simulink model "THEIA_EPS"  (R2024b)
settings: Solver=FixedStepDiscrete  StartTime=0.0  StopTime=60  RelTol=1e-3
undefined symbols (not defined in the file or in its folder): Ion, Lithium
libraries: spsSeriesRLCBranchLib x7, spsIGBTDiodeLib x3, spsIdealSwitchLib x2, slpidlib x2, spsPWMGeneratorDCDCLib x2, spsBatteryLib x1, spsCurrentMeasurementLib x1, spsDiodeLib x1, spsPVArrayLib x1, spsVoltageMeasurementLib x1, sps_lib x1
settings Model: SimulationMode=accelerator  Creator=Josh  LastModifiedBy=Josh

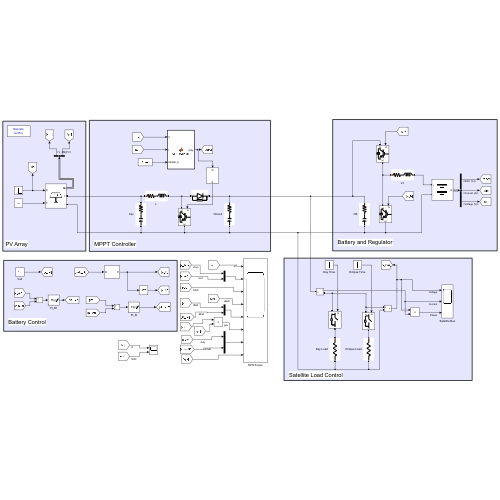
[thumbnail: Simulink's stored preview of the top-level diagram]
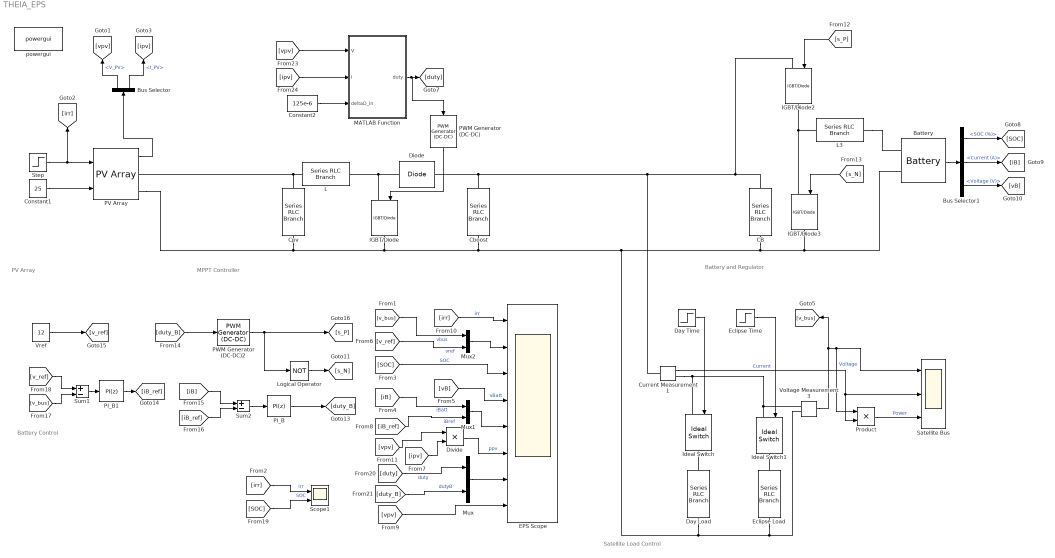
== system THEIA_EPS ==
  note: Battery Control
  note: Satellite Load Control
  note: Battery and Regulator
  note: MPPT Controller
  note: PV Array
  Battery : spsBatteryLib/Battery  BatType=Lithium-Ion  NomV=8  NomQ=12.5  SOC=80  Batt_Tr=1  PresetModel=on  MaxQ=12.5  MinV=6  FullV=9.3119  Dis_rate=5.4348  R=0.0064  Normal_OP=11.3043  expZone="[8.6431     0.61413]"
  Bus Selector : BusSelector  OutputSignals=V_PV,I_PV
  Bus Selector1 : BusSelector  OutputSignals=SOC (%),Current (A),Voltage (V)
  CB : spsSeriesRLCBranchLib/Series RLC Branch  LConnTagsString=__new0  RConnTagsString=__new0  BranchType=RC  Resistance=1e-4  Inductance=1e-3  SetiL0=off  InitialCurrent=0  Capacitance=1000e-6  Setx0=off  InitialVoltage=0  Measurements=None
  Cboost : spsSeriesRLCBranchLib/Series RLC Branch  LConnTagsString=__new0  RConnTagsString=__new0  BranchType=RC  Resistance=1e-4  Inductance=1e-3  SetiL0=off  InitialCurrent=0  Capacitance=3300e-6  Setx0=off  InitialVoltage=0  Measurements=None
  Constant1 : Constant  Value=25
  Constant2 : Constant  Value=125e-6
  Cpv : spsSeriesRLCBranchLib/Series RLC Branch  LConnTagsString=__new0  RConnTagsString=__new0  BranchType=RC  Resistance=1e-4  Inductance=1e-3  SetiL0=off  InitialCurrent=0  Capacitance=100e-6  Setx0=off  InitialVoltage=0  Measurements=None
  Current Measurement1 : spsCurrentMeasurementLib/Current Measurement  PhasorSimulation=off  OutputType=Complex  PSBequivalent=0
  Day Load : spsSeriesRLCBranchLib/Series RLC Branch  LConnTagsString=__new0  RConnTagsString=__new0  BranchType=R  Resistance=1.7  Inductance=5e-3  SetiL0=off  InitialCurrent=0  Capacitance=100e-6  Setx0=off  InitialVoltage=0  Measurements=None
  Day Time : Step  Time=30  Before=1  After=0  SampleTime=0
  Diode : spsDiodeLib/Diode  Ron=0.001  Lon=0  Vf=0.8  IC=0  UseSnubber=0  Rs=5000  Cs=250e-9  Measurements=off
  Divide : Product  Inputs=**
  EPS Scope : Scope  NumInputPorts=8
  Eclipse Load : spsSeriesRLCBranchLib/Series RLC Branch  LConnTagsString=__new0  RConnTagsString=__new0  BranchType=R  Resistance=31  Inductance=5e-3  SetiL0=off  InitialCurrent=0  Capacitance=100e-6  Setx0=off  InitialVoltage=0  Measurements=None
  Eclipse Time : Step  Time=30  SampleTime=0
  IGBT/Diode : spsIGBTDiodeLib/IGBT//Diode  Ron=1e-3  Rs=1e5  Cs=inf  Measurements=off
  IGBT/Diode2 : spsIGBTDiodeLib/IGBT//Diode  Ron=1e-3  Rs=1e5  Cs=inf  Measurements=off
  IGBT/Diode3 : spsIGBTDiodeLib/IGBT//Diode  Ron=1e-3  Rs=1e5  Cs=inf  Measurements=off
  Ideal Switch : spsIdealSwitchLib/Ideal Switch  Ron=0.001  Lon=0  IC=0  Rs=1e5  Cs=inf  Measurements=off
  Ideal Switch1 : spsIdealSwitchLib/Ideal Switch  Ron=0.001  Lon=0  IC=0  Rs=1e5  Cs=inf  Measurements=off
  L : spsSeriesRLCBranchLib/Series RLC Branch  LConnTagsString=__new0  RConnTagsString=__new0  BranchType=RL  Resistance=0.1  Inductance=5e-3  SetiL0=off  InitialCurrent=0  Capacitance=100e-6  Setx0=off  InitialVoltage=0  Measurements=None
  L3 : spsSeriesRLCBranchLib/Series RLC Branch  LConnTagsString=__new0  RConnTagsString=__new0  BranchType=RL  Resistance=0.1  Inductance=5e-3  SetiL0=off  InitialCurrent=0  Capacitance=100e-6  Setx0=off  InitialVoltage=0  Measurements=None
  Logical Operator : Logic  Operator=NOT  AllPortsSameDT=off  OutDataTypeStr=boolean
  MATLAB Function : MATLAB Function  TreatAsAtomicUnit=on
  Mux : Mux  Inputs=2
  Mux1 : Mux  Inputs=2
  Mux2 : Mux  Inputs=2
  PI_B : slpidlib/PID Controller  Controller=PI  Form=Parallel  TimeDomain=Discrete-time  UseExternalTs=off  SampleTime=50e-6  IntegratorMethod=Forward Euler  FilterMethod=Forward Euler  ControllerParametersSource=internal  P=0.02  I=10  UseKiTs=off  D=1e-4  UseExternalDerivativeSource=off  N=100  UseFilter=off  TunerSelectOption=Transfer Function Based (PID Tuner App)  InitialConditionSource=internal  InitialConditionForIntegrator=0  InitialConditionForFilter=0  DifferentiatorICPrevScaledInput=0  ExternalReset=none  TrackingMode=off  Kt=1  LimitOutput=on  SatLimitsSource=internal  UpperSaturationLimit=0.95  LowerSaturationLimit=0  LinearizeAsGain=off  AntiWindupMode=none  Kb=1  LimitIntegrator=off  UpperIntegratorSaturationLimit=inf  LowerIntegratorSaturationLimit=-inf  POutMin=[]  POutMax=[]  IOutMin=[]  IOutMax=[]  DOutMin=[]  DOutMax=[]  NOutMin=[]  NOutMax=[]  SumOutMin=[]  SumOutMax=[]  SaturationOutMin=[]  SaturationOutMax=[]  PParamMin=[]  PParamMax=[]  IParamMin=[]  IParamMax=[]  DParamMin=[]  DParamMax=[]  NParamMin=[]  NParamMax=[]  KbParamMin=[]  KbParamMax=[]  KtParamMin=[]  KtParamMax=[]  KbOutMin=[]  KbOutMax=[]  KtOutMin=[]  KtOutMax=[]  IntegratorOutMin=[]  IntegratorOutMax=[]  FilterOutMin=[]  FilterOutMax=[]  SumI1OutMin=[]  SumI1OutMax=[]  SumI2OutMin=[]  SumI2OutMax=[]  SumI3OutMin=[]  SumI3OutMax=[]  SumI4OutMin=[]  SumI4OutMax=[]  SumDOutMin=[]  SumDOutMax=[]  DifferentiatorOutMin=[]  DifferentiatorOutMax=[]  FilterDiffOutCoefMin=[]  FilterDiffOutCoefMax=[]  ReciprocalOutMin=[]  ReciprocalOutMax=[]  SumDenOutMin=[]  SumDenOutMax=[]  SumNumOutMin=[]  SumNumOutMax=[]  DivideOutMin=[]  DivideOutMax=[]  UdiffTsProdOutMin=[]  UdiffTsProdOutMax=[]  NTsProdOutMin=[]  NTsProdOutMax=[]  UintegralTsProdOutMin=[]  UintegralTsProdOutMax=[]  UngainTsProdOutMin=[]  UngainTsProdOutMax=[]  ClampingZeroOutDataTypeStr=Inherit: Inherit via back propagation  ClampingZeroOutMin=[]  ClampingZeroOutMax=[]  FilterDenConstantOutDataTypeStr=Inherit: Inherit via back propagation  FilterDenConstantOutMin=[]  FilterDenConstantOutMax=[]  PCopyOutDataTypeStr=Inherit: Inherit via back propagation  PCopyOutMin=[]  PCopyOutMax=[]  NCopyOutDataTypeStr=Inherit: Inherit via back propagation  NCopyOutMin=[]  NCopyOutMax=[]  IntegratorContinuousStateAttributes=''  IntegratorStateMustResolveToSignalObject=off  IntegratorRTWStateStorageClass=Auto  FilterContinuousStateAttributes=''  FilterStateMustResolveToSignalObject=off  FilterRTWStateStorageClass=Auto  ParallelPVariant=InternalParameters  IdealPVariant=Disabled  IVariant=InternalParameters  DVariant=Disabled  IntegratorVariant=Discrete  SatVariant=Enabled  AWVariant=Passthrough  PCopyVariant=Disabled  TRVariant=Disabled  FdbkBlocksVariant=Forward  IdealPFdbkVariant=Disabled  SatFdbkVariant=Disabled  DerivativeFilterVariant=Disabled  NVariant=Disabled  NCopyVariant=Disabled_SignalSpec  FilterICVariant=Disabled  IntegratorICVariant=InternalICs  ExternalResetVariant=Disabled  TRSumVariant=Passthrough  SumFdbkVariant=Disabled  SumVariant=Sum_PI  TsampFilterVariant=InternalTs  TsampNgainVariant=Passthrough  TsampIntegralVariant=Disabled_SignalSpec  ExternalSaturationOutDataTypeStr=Inherit: Same as second input  DerivativeSourceVariant=Disabled  PreIntVariant=InternalPreInt
      settings: LibrarySourceBlock=simulink/Discrete/Discrete PID Controller
  PI_B1 : slpidlib/PID Controller  Controller=PI  Form=Parallel  TimeDomain=Discrete-time  UseExternalTs=off  SampleTime=500e-6  IntegratorMethod=Forward Euler  FilterMethod=Forward Euler  ControllerParametersSource=internal  P=0.8  I=5  UseKiTs=off  D=10  UseExternalDerivativeSource=off  N=100  UseFilter=on  TunerSelectOption=Frequency Response Based  InitialConditionSource=internal  InitialConditionForIntegrator=0  InitialConditionForFilter=0  DifferentiatorICPrevScaledInput=0  ExternalReset=none  TrackingMode=off  Kt=1  LimitOutput=on  SatLimitsSource=internal  UpperSaturationLimit=5.5  LowerSaturationLimit=-5.5  LinearizeAsGain=off  AntiWindupMode=none  Kb=1  LimitIntegrator=off  UpperIntegratorSaturationLimit=inf  LowerIntegratorSaturationLimit=-inf  POutMin=[]  POutMax=[]  IOutMin=[]  IOutMax=[]  DOutMin=[]  DOutMax=[]  NOutMin=[]  NOutMax=[]  SumOutMin=[]  SumOutMax=[]  SaturationOutMin=[]  SaturationOutMax=[]  PParamMin=[]  PParamMax=[]  IParamMin=[]  IParamMax=[]  DParamMin=[]  DParamMax=[]  NParamMin=[]  NParamMax=[]  KbParamMin=[]  KbParamMax=[]  KtParamMin=[]  KtParamMax=[]  KbOutMin=[]  KbOutMax=[]  KtOutMin=[]  KtOutMax=[]  IntegratorOutMin=[]  IntegratorOutMax=[]  FilterOutMin=[]  FilterOutMax=[]  SumI1OutMin=[]  SumI1OutMax=[]  SumI2OutMin=[]  SumI2OutMax=[]  SumI3OutMin=[]  SumI3OutMax=[]  SumI4OutMin=[]  SumI4OutMax=[]  SumDOutMin=[]  SumDOutMax=[]  DifferentiatorOutMin=[]  DifferentiatorOutMax=[]  FilterDiffOutCoefMin=[]  FilterDiffOutCoefMax=[]  ReciprocalOutMin=[]  ReciprocalOutMax=[]  SumDenOutMin=[]  SumDenOutMax=[]  SumNumOutMin=[]  SumNumOutMax=[]  DivideOutMin=[]  DivideOutMax=[]  UdiffTsProdOutMin=[]  UdiffTsProdOutMax=[]  NTsProdOutMin=[]  NTsProdOutMax=[]  UintegralTsProdOutMin=[]  UintegralTsProdOutMax=[]  UngainTsProdOutMin=[]  UngainTsProdOutMax=[]  ClampingZeroOutDataTypeStr=Inherit: Inherit via back propagation  ClampingZeroOutMin=[]  ClampingZeroOutMax=[]  FilterDenConstantOutDataTypeStr=Inherit: Inherit via back propagation  FilterDenConstantOutMin=[]  FilterDenConstantOutMax=[]  PCopyOutDataTypeStr=Inherit: Inherit via back propagation  PCopyOutMin=[]  PCopyOutMax=[]  NCopyOutDataTypeStr=Inherit: Inherit via back propagation  NCopyOutMin=[]  NCopyOutMax=[]  IntegratorContinuousStateAttributes=''  IntegratorStateMustResolveToSignalObject=off  IntegratorRTWStateStorageClass=Auto  FilterContinuousStateAttributes=''  FilterStateMustResolveToSignalObject=off  FilterRTWStateStorageClass=Auto  ParallelPVariant=InternalParameters  IdealPVariant=Disabled  IVariant=InternalParameters  DVariant=Disabled  IntegratorVariant=Discrete  SatVariant=Enabled  AWVariant=Passthrough  PCopyVariant=Disabled  TRVariant=Disabled  FdbkBlocksVariant=Forward  IdealPFdbkVariant=Disabled  SatFdbkVariant=Disabled  DerivativeFilterVariant=Disabled  NVariant=Disabled  NCopyVariant=Disabled_SignalSpec  FilterICVariant=Disabled  IntegratorICVariant=InternalICs  ExternalResetVariant=Disabled  TRSumVariant=Passthrough  SumFdbkVariant=Disabled  SumVariant=Sum_PI  TsampFilterVariant=InternalTs  TsampNgainVariant=Passthrough  TsampIntegralVariant=Disabled_SignalSpec  ExternalSaturationOutDataTypeStr=Inherit: Same as second input  DerivativeSourceVariant=Disabled  PreIntVariant=InternalPreInt
      settings: LibrarySourceBlock=simulink/Discrete/Discrete PID Controller
  PV Array : spsPVArrayLib/PV Array  Npar=18  Nser=1  PlotType=array @ 25 deg.C & specified irradiances  S_vec=[1367 1000 500 0]  Temp_C_vec="[ 45 25  ]"  ModuleName=User-defined  PlotWhenSelected=off  Pm=5.0021  Ncell=7  Voc=17.136  Isc=0.342  Vm=15.1578  Im=0.33  beta_Voc_pc=-0.2369  alpha_Isc_pc=0.0022  beta_Voc=-0.040595  alpha_Isc=7.524e-06  IL=0.34471  I0=5.8844e-14  nI=3.2418  Rsh=7127.5853  Rs=0.16891  RobustModel=off  RobustCellTemperature=313.3991  BAL=on  Tc=1e-6  Tfilter=5e-5
  PWM Generator (DC-DC) : spsPWMGeneratorDCDCLib/PWM Generator (DC-DC)  Fsw=5000  Ts=10e-6
  PWM Generator (DC-DC)2 : spsPWMGeneratorDCDCLib/PWM Generator (DC-DC)  Fsw=5000  Ts=10e-6
  Product : Product
  Satellite Bus : Scope  NumInputPorts=3
  Scope1 : Scope  NumInputPorts=2
  Step : Step  Time=30  Before=1367  After=0  SampleTime=0
  Sum1 : Sum  Inputs=+-
  Sum2 : Sum  Inputs=+-
  Voltage Measurement3 : spsVoltageMeasurementLib/Voltage Measurement  PhasorSimulation=off  OutputType=Complex  PSBequivalent=0
  Vref : Constant  Value=12
  powergui : sps_lib/powergui  Priority=1  SimulationMode=Discrete  SampleTime=10e-6  frequency=60  Iterations=50  frequencyindice=0  Pbase=100e6  ErrMax=1e-4  UnitsV=kV  UnitsW=MW  buscounter=0  FunctionMessages=off  echomessages=off  EnableUseOfTLC=off  CurrentSourceSwitches=off  DisableSnubberDevices=off  DisableRonSwitches=off  DisableVfSwitches=off  DisplayEquations=off  AutomaticDiscreteSolvers=off  SolverType=Tustin/Backward Euler (TBE)  Interpol=off  ExternalGateDelay=off  methode=off  Ts=100  x0status=blocks  SPID=on  SwTol=0  HookPort=off  NonlinearTolerance=1e-4  nMaxIteration=100  ContinueOnMaxIteration=off  RestoreLinks=warning  ResistiveCurrentMeasurement=off  Frange=[0:2:500]  Ylog=off  Xlog=on  ShowGrid=off  save=off  variable=ZData  structure=0  ZoomFFT=off  StartTime=0.0  cycles=1  DisplayStyle=1  fundamental=60  FreqAxis=off  MaxFrequency=1000  frequencyindicesteady=1  RmsSteady=1  display=off
  wires:
  Constant1/1 -> PV Array/2
  Step/1 -> [irr], PV Array/1
  Constant2/1 -> MATLAB Function/3(deltaD_in)
  MATLAB Function/1(duty) -> PWM Generator (DC-DC)/1, [duty]
  PWM Generator (DC-DC)/1 -> IGBT/Diode/1
  PWM Generator (DC-DC)2/1 -> Logical Operator/1, [s_P]
  Sum2/1 -> PI_B/1
  Vref/1 -> [v_ref]
  PI_B1/1 -> [iB_ref]
  [duty_B] -> PWM Generator (DC-DC)2/1
  PI_B/1 -> [duty_B]
  Sum1/1 -> PI_B1/1
  [s_P] -> IGBT/Diode2/1
  Battery/1 -> Bus Selector1/1
  [s_N] -> IGBT/Diode3/1
  Bus Selector1/1 -> [SOC]  "<SOC (%)>"
  Bus Selector1/2 -> [iB]  "<Current (A)>"
  Bus Selector1/3 -> [vB]  "<Voltage (V)>"
  [vB] -> EPS Scope/4  "vBatt"
  [irr] -> EPS Scope/1  "irr"
  Mux1/1 -> EPS Scope/5
  [iB] -> Mux1/1  "iBatt"
  [iB_ref] -> Mux1/2  "iBref"
  Mux2/1 -> EPS Scope/2
  [v_bus] -> Mux2/1  "vbus"
  [v_ref] -> Mux2/2  "vref"
  [SOC] -> EPS Scope/3  "SOC"
  [ipv] -> Divide/2
  [vpv] -> Divide/1
  Divide/1 -> EPS Scope/6  "ppv"
  PV Array/1 -> Bus Selector/1
  Bus Selector/2 -> [ipv]  "<I_PV>"
  Bus Selector/1 -> [vpv]  "<V_PV>"
  Mux/1 -> EPS Scope/7
  [duty] -> Mux/1  "duty"
  [duty_B] -> Mux/2  "dutyB"
  [v_ref] -> Sum1/1
  [v_bus] -> Sum1/2
  [vpv] -> EPS Scope/8
  Voltage Measurement3/1 -> [v_bus], Product/1, Satellite Bus/1  "Voltage"
  Current Measurement1/1 -> Product/2, Satellite Bus/2  "Current"
  Product/1 -> Satellite Bus/3  "Power"
  Day Time/1 -> Ideal Switch/1
  Eclipse Time/1 -> Ideal Switch1/1
  [vpv] -> MATLAB Function/1(V)
  [ipv] -> MATLAB Function/2(I)
  [iB] -> Sum2/1
  [iB_ref] -> Sum2/2
  Logical Operator/1 -> [s_N]
  [irr] -> Scope1/1  "irr"
  [SOC] -> Scope1/2  "SOC"
  connections:
  Cpv/LConn1 -- PV Array/RConn1 -- L/LConn1
  IGBT/Diode/LConn1 -- Diode/LConn1 -- L/RConn1
  L3/LConn1 -- IGBT/Diode2/RConn1 -- IGBT/Diode3/LConn1
  L3/RConn1 -- Battery/LConn1
  Day Load/LConn1 -- Ideal Switch/RConn1
  Eclipse Load/LConn1 -- Ideal Switch1/RConn1
  Current Measurement1/RConn1 -- Ideal Switch1/LConn1 -- Voltage Measurement3/LConn1 -- Ideal Switch/LConn1
  Diode/RConn1 -- CB/LConn1 -- IGBT/Diode2/LConn1 -- Current Measurement1/LConn1 -- Cboost/LConn1
  IGBT/Diode/RConn1 -- Cboost/RConn1 -- CB/RConn1 -- Battery/LConn2 -- IGBT/Diode3/RConn1 -- Voltage Measurement3/LConn2 -- Eclipse Load/RConn1 -- Day Load/RConn1 -- PV Array/RConn2 -- Cpv/RConn1

== matlab function THEIA_EPS/MATLAB Function ==
  data: V input; duty output; I input; deltaD_in input
function duty = MPPTControl(V, I, deltaD_in)

duty_init = 0.05;
duty_min = 0;
duty_max = 0.85;

persistent Vold Pold duty_old;

if isempty(Vold)
    Vold = 0;
    Pold = 0;
    duty_old = duty_init;
end

P = V*I;
dV = V - Vold;
dP = P - Pold;
duty = duty_old;
deltaD = deltaD_in;

if dP ~= 0
    if dP < 0
        if dV < 0
            duty = duty_old - deltaD;
        else
            duty = duty_old + deltaD;
        end
    else
        if dV > 0
            duty = duty_old + deltaD;
        else
            duty = duty_old - deltaD;
        end
    end
end

if duty >= duty_max
    duty = duty_max;
elseif duty < duty_min
    duty = duty_min;
end

duty_old = duty;
Vold = V;
Pold = P;

end
